simulink model "simulinkmodel"  (R2021a)
settings: Solver=VariableStepAuto  StartTime=0.0  StopTime=10.0  RelTol=1e-3
values from neighbouring files (symbols this model uses):
  g = 9.81    [pid_parameters.m]
  I = 0.00017701    [pid_parameters.m]
  M = 0.703    [pid_parameters.m]
  m = 0.024    [pid_parameters.m]
undefined symbols (not defined in the file or in its folder): L
settings Model: Creator=ryusei  LastModifiedBy=ryusei

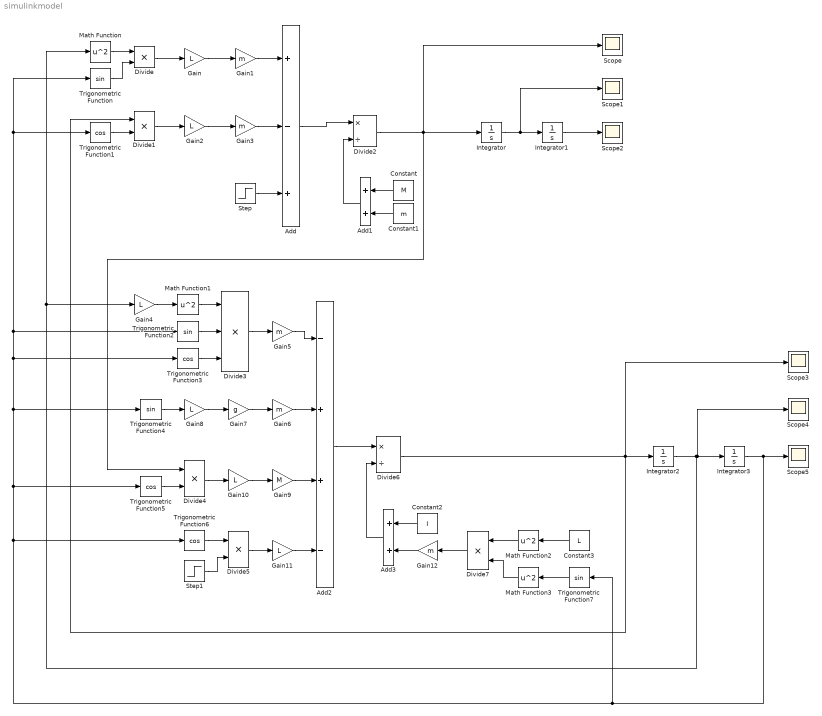
== system simulinkmodel ==
  Add : Sum  Inputs=+-+
  Add1 : Sum
  Add2 : Sum  Inputs=-++-
  Add3 : Sum
  Constant : Constant  Value=M
  Constant1 : Constant  Value=m
  Constant2 : Constant  Value=I
  Constant3 : Constant  Value=L
  Divide{,1,4..5,7} (5 alike) : Product  Inputs=**
  Divide2 : Product  Inputs=*/
  Divide3 : Product  Inputs=***
  Divide6 : Product  Inputs=*/
  Gain{,2,4,8,10..11} (6 alike) : Gain  Gain=L
  Gain{1,3,5..6,12} (5 alike) : Gain  Gain=m
  Gain7 : Gain  Gain=g
  Gain9 : Gain  Gain=M
  Integrator{,1..3} (4 alike) : Integrator
  Math Function{,1..3} (4 alike) : Math  Operator=square  SaturateOnIntegerOverflow=on
  Scope{,1..5} (6 alike) : Scope
  Step : Step  SampleTime=0
  Step1 : Step  SampleTime=0
  Trigonometric Function{,2,4,7} (4 alike) : Trigonometry
  Trigonometric Function{1,3,5..6} (4 alike) : Trigonometry  Operator=cos
  wires:
  Math Function/1 -> Divide/1
  Divide/1 -> Gain/1
  Gain/1 -> Gain1/1
  Trigonometric Function/1 -> Divide/2
  Gain1/1 -> Add/1
  Trigonometric Function1/1 -> Divide1/2
  Divide1/1 -> Gain2/1
  Gain2/1 -> Gain3/1
  Gain3/1 -> Add/2
  Step/1 -> Add/3
  Add/1 -> Divide2/1
  Add1/1 -> Divide2/2
  Constant/1 -> Add1/1
  Constant1/1 -> Add1/2
  Integrator/1 -> Scope1/1, Integrator1/1
  Integrator1/1 -> Scope2/1
  Gain4/1 -> Math Function1/1
  Math Function1/1 -> Divide3/1
  Trigonometric Function2/1 -> Divide3/2
  Trigonometric Function3/1 -> Divide3/3
  Divide3/1 -> Gain5/1
  Trigonometric Function4/1 -> Gain8/1
  Gain8/1 -> Gain7/1
  Gain7/1 -> Gain6/1
  Gain6/1 -> Add2/2
  Divide4/1 -> Gain10/1
  Gain10/1 -> Gain9/1
  Gain9/1 -> Add2/3
  Trigonometric Function5/1 -> Divide4/2
  Trigonometric Function6/1 -> Divide5/1
  Step1/1 -> Divide5/2
  Divide5/1 -> Gain11/1
  Gain11/1 -> Add2/4
  Add2/1 -> Divide6/1
  Gain5/1 -> Add2/1
  Constant2/1 -> Add3/1
  Gain12/1 -> Add3/2
  Divide7/1 -> Gain12/1
  Math Function2/1 -> Divide7/1
  Constant3/1 -> Math Function2/1
  Math Function3/1 -> Divide7/2
  Trigonometric Function7/1 -> Math Function3/1
  Add3/1 -> Divide6/2
  Divide2/1 -> Scope/1, Divide4/1, Integrator/1
  Integrator2/1 -> Gain4/1, Math Function/1, Scope4/1, Integrator3/1
  Divide6/1 -> Scope3/1, Divide1/1, Integrator2/1
  Integrator3/1 -> Scope5/1, Trigonometric Function7/1, Trigonometric Function5/1, Trigonometric Function4/1, Trigonometric Function3/1, Trigonometric Function2/1, Trigonometric Function1/1, Trigonometric Function/1, Trigonometric Function6/1
